simulink model "essescalon"  (R2014a)
settings: Solver=ode45  StartTime=0.0  StopTime=30  RelTol=1e-3
settings Model: Creator=Nury  LastModifiedBy=Nury
settings DebuggingCC: SolverPrmCheckMsg=none

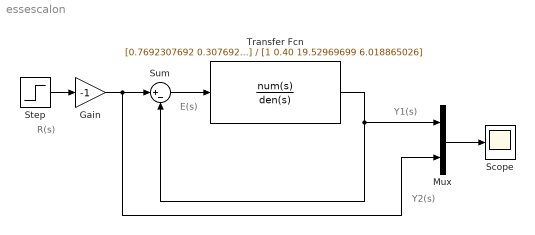
== system essescalon ==
  note: Y2(s)
  note: Y1(s)
  note: R(s)
  note: E(s)
  Gain : Gain  Gain=-1
  Mux : Mux  Inputs=2
  Scope : Scope
  Step : Step  Before=1
  Sum : Sum  Inputs=|+-
  Transfer Fcn : TransferFcn  Numerator=[0.7692307692 0.3076923077 15.02284384]  Denominator=[1 0.40 19.52969699 6.018865026]
  wires:
  Sum/1 -> Transfer Fcn/1
  Mux/1 -> Scope/1
  Transfer Fcn/1 -> Sum/2, Mux/1
  Gain/1 -> Mux/2, Sum/1
  Step/1 -> Gain/1
